simulink model "Mission_Supervisor_1drone_insideCP"  (R2019b)
settings: Solver=FixedStepAuto  StartTime=0.0  StopTime=inf  FixedStep=0.025  RelTol=1e-3  EnableMultiTasking=on
InitFcn:
  | global clientID;
  | clientID=-1;
libraries: dspindex x4
settings Model: EnablePacing=on  Creator=Kleber Cabral  LastModifiedBy=Kleber Cabral
settings DataIOCC: SaveFormat=Array  ReturnWorkspaceOutputs=off
settings OptimizationCC: LifeSpan=inf
settings DebuggingCC: SolverPrmCheckMsg=warning  SFUnexpectedBacktrackingDiag=warning  SFNoUnconditionalDefaultTransitionDiag=warning  ArithmeticOperatorsInVariantConditions=warning
settings HardwareCC: ProdBitPerPointer=32  ProdBitPerSizeT=32  ProdBitPerPtrDiffT=32  ProdLargestAtomicFloat=None  ProdIntDivRoundTo=Undefined  ProdEndianess=Unspecified  ProdWordSize=32  ProdHWDeviceType=32-bit Generic
settings ModelReferenceCC: PropagateSignalLabelsOutOfModel=off
settings SFSimCC: SimUseLocalCustomCode=off  CustomCodeUndefinedFunction=UseInterfaceOnly
settings RTWCC: RTWUseLocalCustomCode=off
settings CodeAppCC: StateflowObjectComments=on
settings GRTTargetCC: TargetLangStandard=C89/C90 (ANSI)  GeneratePreprocessorConditionals=Disable all
settings ConfigComp: CovMetricSettings=dw  CovHtmlReporting=on  CovSaveCumulativeToWorkspaceVar=on  CovSaveSingleToWorkspaceVar=on  CovExternalEMLEnable=off  CovSFcnEnable=off

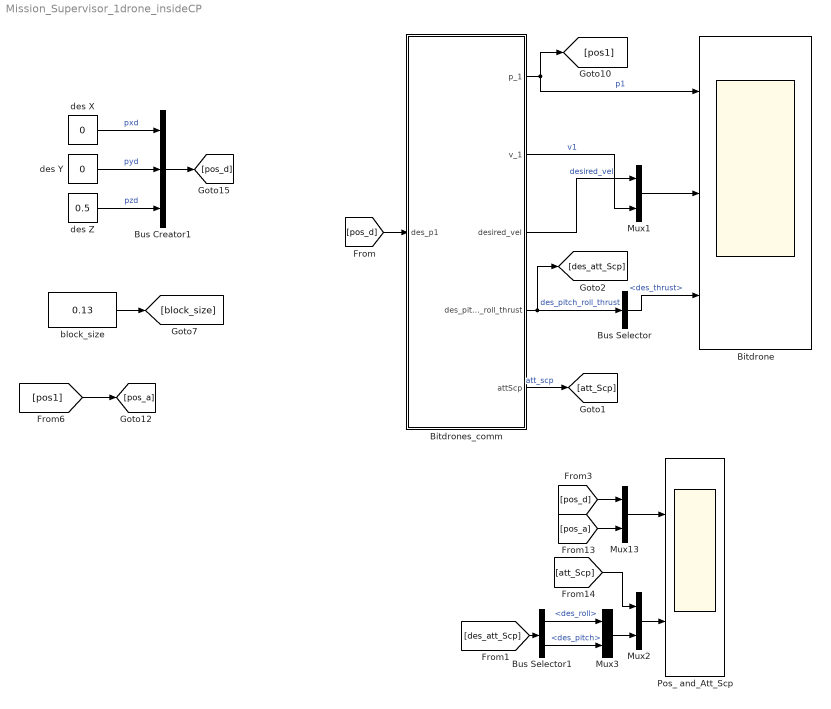
== system Mission_Supervisor_1drone_insideCP ==
  Bitdrone : Scope  NumInputPorts=3
  Bitdrones_comm : Subsystem
  Bus Creator1 : BusCreator  Inputs=3
  Bus Selector : BusSelector  OutputSignals=des_thrust
  Bus Selector1 : BusSelector  OutputSignals=des_roll,des_pitch
  Mux{1..3,13} (4 alike) : Mux  Inputs=2
  Pos_ and_Att_Scp : Scope  NumInputPorts=2
  block_size : Constant  Value=0.13
  des X : Constant  Value=0
  des Y : Constant  Value=0
  des Z : Constant  Value=0.5
  wires:
  des X/1 -> Bus Creator1/1  "pxd"
  des Y/1 -> Bus Creator1/2  "pyd"
  des Z/1 -> Bus Creator1/3  "pzd"
  block_size/1 -> [block_size]
  Bitdrones_comm/2(v_1) -> Mux1/2  "v1"
  Bitdrones_comm/1(p_1) -> [pos1], Bitdrone/1  "p1"
  Bitdrones_comm/3(desired_vel) -> Mux1/1  "desired_vel"
  Bitdrones_comm/5(attScp) -> [att_Scp]  "att_scp"
  [att_Scp] -> Mux2/1
  [pos_d] -> Mux13/1
  Mux13/1 -> Pos_ and_Att_Scp/1
  [pos_a] -> Mux13/2
  Bus Creator1/1 -> [pos_d]
  [pos_d] -> Bitdrones_comm/1(des_p1)
  [pos1] -> [pos_a]
  Mux1/1 -> Bitdrone/2
  Bitdrones_comm/4(des_pitch_roll_thrust) -> [des_att_Scp], Bus Selector/1  "des_pitch_roll_thrust"
  Bus Selector/1 -> Bitdrone/3  "<des_thrust>"
  [des_att_Scp] -> Bus Selector1/1
  Bus Selector1/2 -> Mux3/2  "<des_pitch>"
  Bus Selector1/1 -> Mux3/1  "<des_roll>"
  Mux3/1 -> Mux2/2
  Mux2/1 -> Pos_ and_Att_Scp/2

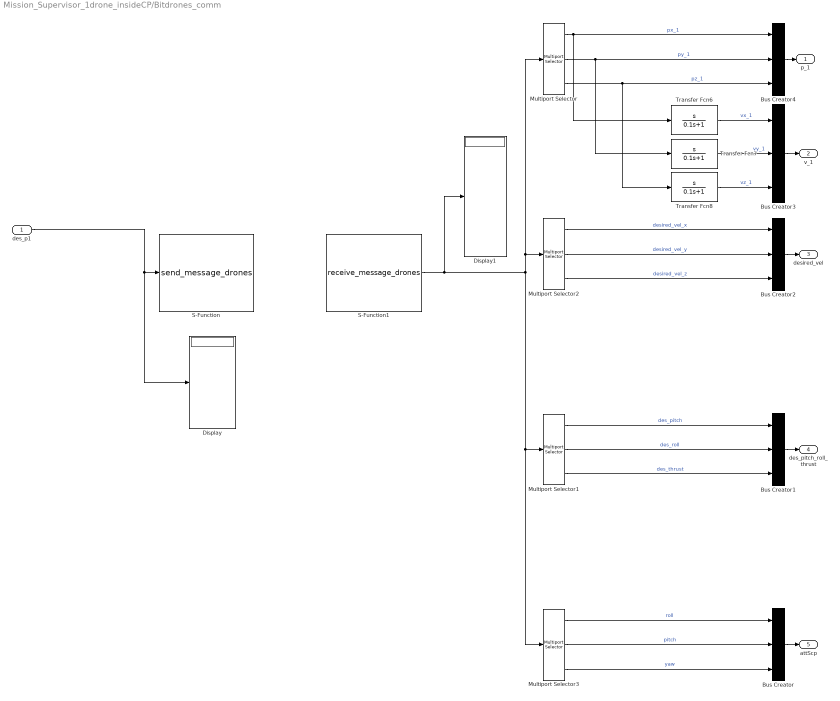
== system Mission_Supervisor_1drone_insideCP/Bitdrones_comm ==
  des_p1 : Inport
  Bus Creator{,1..4} (5 alike) : BusCreator  Inputs=3
  Display : Display
      settings: Decimation=3
  Display1 : Display
      settings: Decimation=3
  Multiport Selector : dspindex/Multiport Selector  rowsOrCols=Rows  idxCellArray={1,2,3}  idxErrMode=Clip Index
  Multiport Selector1 : dspindex/Multiport Selector  rowsOrCols=Rows  idxCellArray={7,8,9}  idxErrMode=Clip Index
  Multiport Selector2 : dspindex/Multiport Selector  rowsOrCols=Rows  idxCellArray={4,5,6}  idxErrMode=Clip Index
  Multiport Selector3 : dspindex/Multiport Selector  rowsOrCols=Rows  idxCellArray={10,11,12}  idxErrMode=Clip Index
  S-Function : S-Function  FunctionName=send_message_drones  SFunctionDeploymentMode=off  EnableBusSupport=off
  S-Function1 : S-Function  FunctionName=receive_message_drones  SFunctionDeploymentMode=off  EnableBusSupport=off
  Transfer Fcn6 : TransferFcn  Numerator=[1 0]  Denominator=[0.1 1]
  Transfer Fcn7 : TransferFcn  Numerator=[1 0]  Denominator=[0.1 1]
  Transfer Fcn8 : TransferFcn  Numerator=[1 0]  Denominator=[0.1 1]
  p_1 : Outport
  v_1 : Outport  Port=2
  desired_vel : Outport  Port=3
  des_pitch_roll_thrust : Outport  Port=4
  attScp : Outport  Port=5
  wires:
  Multiport Selector/1 -> Bus Creator4/1, Transfer Fcn6/1  "px_1"
  Multiport Selector/2 -> Bus Creator4/2, Transfer Fcn7/1  "py_1"
  Multiport Selector/3 -> Bus Creator4/3, Transfer Fcn8/1  "pz_1"
  Multiport Selector2/1 -> Bus Creator2/1  "desired_vel_x"
  Multiport Selector2/2 -> Bus Creator2/2  "desired_vel_y"
  Multiport Selector2/3 -> Bus Creator2/3  "desired_vel_z"
  des_p1/1 -> Display/1, S-Function/1
  Bus Creator4/1 -> p_1/1
  Bus Creator2/1 -> desired_vel/1
  Transfer Fcn6/1 -> Bus Creator3/1  "vx_1"
  Bus Creator3/1 -> v_1/1
  Transfer Fcn8/1 -> Bus Creator3/3  "vz_1"
  Transfer Fcn7/1 -> Bus Creator3/2  "vy_1"
  Bus Creator1/1 -> des_pitch_roll_thrust/1
  Multiport Selector1/2 -> Bus Creator1/2  "des_roll"
  Multiport Selector1/1 -> Bus Creator1/1  "des_pitch"
  Multiport Selector3/2 -> Bus Creator/2  "pitch"
  Multiport Selector3/3 -> Bus Creator/3  "yaw"
  Bus Creator/1 -> attScp/1
  S-Function1/1 -> Display1/1, Multiport Selector/1, Multiport Selector2/1, Multiport Selector3/1, Multiport Selector1/1
  Multiport Selector3/1 -> Bus Creator/1  "roll"
  Multiport Selector1/3 -> Bus Creator1/3  "des_thrust"
